simulink model "HighwayLaneChangeTestBench"  (R2022a)
settings: Solver=VariableStepAuto  StartTime=0.0  StopTime=inf  FixedStep=Ts  RelTol=1e-3
PostLoadFcn:
  | helperSLHighwayLaneChangeSetup;
undefined symbols (not defined in the file): actorProfiles, camera, DiscIntNeverNeededParam, driving, egoFrontExt, egoTTC, enableCCBehavior, enableLCBehavior, enableLCFBehavior, frontSafetyGap, latDevCost, mapInfo, matlabshared, maxAccel, maxCurvature, maxPlanningHorizon, maxYawRate, minVelocity, nextTTC, predictionHorizon, preferredLane, rearSafetyGap, replanRate, scenario, setSpeed, speedCost, targetFrontExt, timeCost, timeHorizon, timeResolution, Ts, u_max, u_min
libraries: drivingscenarioandsensors x8, rllib x1, sensorinslib x1, simulink x1
CloseFcn:
  | helperSLHighwayLaneChangeCleanUp;
settings Model: Creator=The MathWorks, Inc.  LastModifiedBy=leeju
settings SolverCC: ZeroCrossAlgorithm=Adaptive  AlgebraicLoopSolver=TrustRegion  MaxZcPerStep=1
settings DataIOCC: SaveOutput=off
settings DebuggingCC: MaskedZcDiagnostic=none  IgnoredZcDiagnostic=none  UnconnectedInputMsg=warning  UnconnectedOutputMsg=warning  UnconnectedLineMsg=warning  BusObjectLabelMismatch=none  SFMachineParentedDataDiag=warning
settings RTWCC: DLArmComputeVersion=19.05

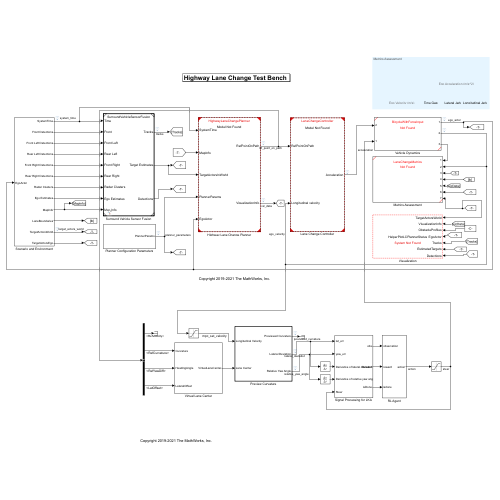
[thumbnail: Simulink's stored preview of the top-level diagram]
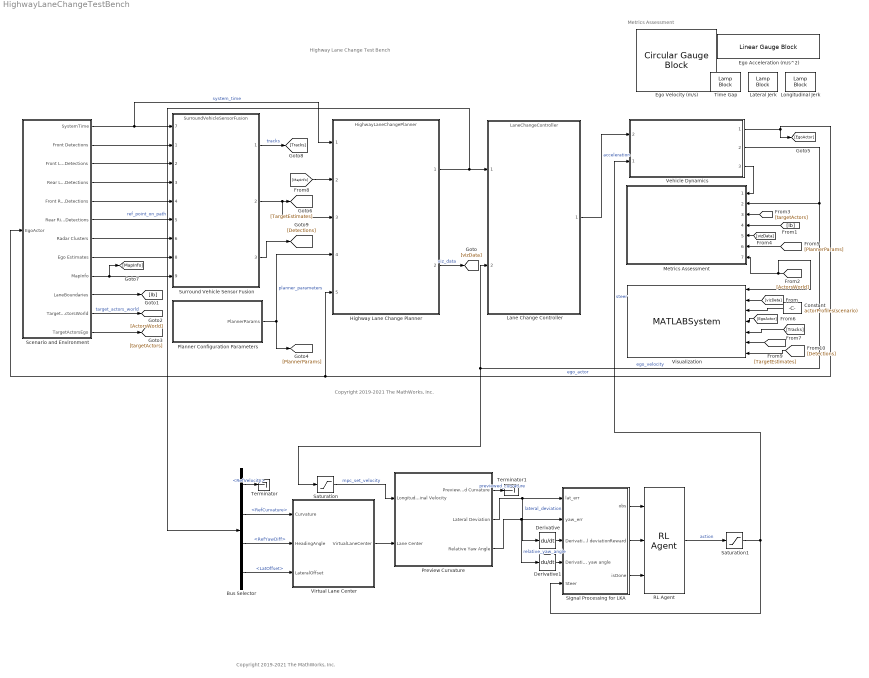
== system HighwayLaneChangeTestBench ==
  note: Copyright 2019-2021 The MathWorks, Inc.
  note: Metrics Assessment
  note: Highway Lane Change Test Bench
  note: Copyright 2019-2021 The MathWorks, Inc.
  Bus Selector : BusSelector  OutputSignals=RefVelocity,RefCurvature,RefYawDiff,LatOffset
  Constant : Constant  Value=actorProfiles(scenario)  OutDataTypeStr=Bus: BusActorProfiles
  Derivative : Derivative
  Derivative1 : Derivative
  Ego Acceleration (m/s^2) : LinearGaugeBlock  LabelPosition=Hide  ScaleMin=-5  ScaleMax=5
  Ego Velocity (m/s) : CircularGaugeBlock  LabelPosition=Hide  ScaleMax=50  TickInterval=5
  Highway Lane Change Planner : ModelReference  ModelNameDialog=HighwayLaneChangePlanner.slx  SimulationMode=Normal  ModelReferenceVersion=5.16
  Lane Change Controller : ModelReference  ModelNameDialog=LaneChangeController.slx  SimulationMode=Normal  ModelReferenceVersion=4.4
  Lateral Jerk : LampBlock  LabelPosition=Hide
  Longitudinal Jerk : LampBlock  LabelPosition=Hide
  Metrics Assessment : Subsystem  ReferencedSubsystem=LaneChangeMetrics
  Planner Configuration Parameters : Subsystem
  Preview Curvature : Subsystem  TreatAsAtomicUnit=on
  RL Agent : rllib/RL Agent  Agent=agent  ExternalActionAsInput=off  ProvideLastAction=off  ProvideCumRwd=off  TreatAsDirectFeedthrough=on  UseStrictObservationDataTypes=off
  Saturation : Saturate  UpperLimit=inf  LowerLimit=0.0001
  Saturation1 : Saturate  UpperLimit=u_max  LowerLimit=u_min
  Scenario and Environment : Subsystem
  "Signal Processing for LKA " : Subsystem
  Surround Vehicle Sensor Fusion : ModelReference  ModelNameDialog=SurroundVehicleSensorFusion.slx  SimulationMode=Normal  ModelReferenceVersion=5.215
      settings: PortSchema="{\"entries\":[{\"content\":{\"sides\":[{\"content\":{\"connectorIds\":[\"In7\",\"In1\",\"In2\",\"In3\",\"In4\",\"In5\",\"In6\",\"In8\",\"In9\"]},\"type\":\"ConnectorPlacement.EquallySpacedRectSide\",\"uuid\":\"babc32b8-473b-4a04-b824-251f7900e603\"},{\"content\":{\"connectorIds\":[\"Out1\",\"Out2\",\"Out3\"],\"side\":\"RIGHT\"},\"type\":\"ConnectorPlacement.EquallySpacedRectSide\",\"uuid\":\"6521796d-8396-47d7-a507-be3f8604ea95\"},{\"content\":{\"connectorIds\":[],\"side\":\"TOP\"},\"type\":\"ConnectorPlacement.EquallySpacedRectSide\",\"uuid\":\"3afcd3a1-01f6-437b-a186-b4f18cfd5e31\"}]},\"type\":\"ConnectorPlacement.EquallySpacedConnector\",\"uuid\":\"2716b65b-56e0-49c3-bc67-2edcf12b2a8e\"}],\"packageUris\":[\"http://schema.mathworks.com/mf0/Connector/R2020b\"],\"version\":\"1.0\"}"
  Terminator : Terminator
  Terminator1 : Terminator
  Time Gap : LampBlock  LabelPosition=Hide
  Vehicle Dynamics : Subsystem  ReferencedSubsystem=BicycleWithForceInput
      settings: PortSchema="{\"entries\":[{\"content\":{\"sides\":[{\"content\":{\"connectorIds\":[\"In2\",\"In1\"]},\"type\":\"ConnectorPlacement.EquallySpacedRectSide\",\"uuid\":\"f63f66bc-f59a-4e63-885b-0681004bade6\"},{\"content\":{\"connectorIds\":[\"Out1\",\"Out2\",\"Out3\"],\"side\":\"RIGHT\"},\"type\":\"ConnectorPlacement.EquallySpacedRectSide\",\"uuid\":\"8ac8ea57-0210-4a13-ad95-4f0a9335ab33\"},{\"content\":{\"connectorIds\":[],\"side\":\"TOP\"},\"type\":\"ConnectorPlacement.EquallySpacedRectSide\",\"uuid\":\"6d0b300d-41b2-47ad-8d2f-35db0d33cdc5\"}]},\"type\":\"ConnectorPlacement.EquallySpacedConnector\",\"uuid\":\"3215dd89-c688-4582-a904-15ea546ef61a\"}],\"packageUris\":[\"http://schema.mathworks.com/mf0/Connector/R2020b\"],\"version\":\"1.0\"}"
  Virtual Lane Center : Subsystem
  Visualization : MATLABSystem  System=HelperPlotLCPlannerStatus  ActorsInfo=Tracks  EnableTopView=on  EnableTrajTopView=on  EnableTracksTopView=on  EnableChaseView=on  EnableTrajChase=on  EnableCaplistChaseView=on  EnableTracksChaseView=on
      mask Type: HelperPlotLCPlannerStatus
      mask Display:
      | disp('HelperPlotLCPlannerStatus');
      | port_label('input',1,'TargetActorsWorld');
      | port_label('input',2,'VisualizationInfo');
      | port_label('input',3,'ObstacleProfiles');
      | port_label('input',4,'EgoActor');
      | port_label('input',5,'Tracks');
      | port_label('input',6,'EstimatedTargets');
      | port_label('input',7,'Detections');
  wires:
  Planner Configuration Parameters/1(PlannerParams) -> Highway Lane Change Planner/4, [PlannerParams]  "planner_parameters"
  Highway Lane Change Planner/2 -> [vizData]  "viz_data"
  Scenario and Environment/10(LaneBoundaries) -> [lb]
  [lb] -> Metrics Assessment/4
  Highway Lane Change Planner/1 -> Bus Selector/1, Lane Change Controller/1  "ref_point_on_path"
  [ActorsWorld] -> Metrics Assessment/7, Visualization/1
  Scenario and Environment/11(TargetActorsWorld) -> [ActorsWorld]  "target_actors_world"
  Scenario and Environment/12(TargetActorsEgo) -> [targetActors]
  [targetActors] -> Metrics Assessment/3
  Scenario and Environment/1(SystemTime) -> Highway Lane Change Planner/1, Surround Vehicle Sensor Fusion/7  "system_time"
  Vehicle Dynamics/1 -> Scenario and Environment/1(EgoActor), Highway Lane Change Planner/5, [EgoActor]  "ego_actor"
  Vehicle Dynamics/2 -> Saturation/1, Lane Change Controller/2, Metrics Assessment/2  "ego_velocity"
  Vehicle Dynamics/3 -> Metrics Assessment/1
  Lane Change Controller/1 -> Vehicle Dynamics/2  "acceleration"
  [vizData] -> Metrics Assessment/5
  [PlannerParams] -> Metrics Assessment/6
  Scenario and Environment/2(Front Detections) -> Surround Vehicle Sensor Fusion/1
  Scenario and Environment/3(Front Left Detections) -> Surround Vehicle Sensor Fusion/2
  Scenario and Environment/4(" Rear Left Detections") -> Surround Vehicle Sensor Fusion/3
  Scenario and Environment/5(Front Right Detections) -> Surround Vehicle Sensor Fusion/4
  Scenario and Environment/6(Rear Right Detections) -> Surround Vehicle Sensor Fusion/5
  Scenario and Environment/7(Radar Clusters) -> Surround Vehicle Sensor Fusion/6
  Scenario and Environment/8(Ego Estimates) -> Surround Vehicle Sensor Fusion/8
  [vizData] -> Visualization/2
  Constant/1 -> Visualization/3
  Scenario and Environment/9(MapInfo) -> Surround Vehicle Sensor Fusion/9, [MapInfo]
  [MapInfo] -> Highway Lane Change Planner/2
  Surround Vehicle Sensor Fusion/2 -> Highway Lane Change Planner/3, [TargetEstimates]
  Surround Vehicle Sensor Fusion/1 -> [Tracks]  "tracks"
  Surround Vehicle Sensor Fusion/3 -> [Detections]
  [Tracks] -> Visualization/5
  [Detections] -> Visualization/7
  [EgoActor] -> Visualization/4
  [TargetEstimates] -> Visualization/6
  Saturation1/1 -> "Signal Processing for LKA "/5(Steer), Vehicle Dynamics/1  "steer"
  Derivative1/1 -> "Signal Processing for LKA "/4(Derivative of relative yaw angle)
  "Signal Processing for LKA "/3(isDone) -> RL Agent/3
  "Signal Processing for LKA "/1(obs) -> RL Agent/1
  RL Agent/1 -> Saturation1/1  "action"
  "Signal Processing for LKA "/2(Reward) -> RL Agent/2
  Bus Selector/3 -> Virtual Lane Center/2(HeadingAngle)  "<RefYawDiff>"
  Saturation/1 -> Preview Curvature/1(Longitudinal Velocity)  "mpc_set_velocity"
  Virtual Lane Center/1(VirtualLaneCenter) -> Preview Curvature/2(Lane Center)
  Preview Curvature/3(Relative Yaw Angle) -> "Signal Processing for LKA "/2(yaw_err), Derivative1/1  "relative_yaw_angle"
  Bus Selector/2 -> Virtual Lane Center/1(Curvature)  "<RefCurvature>"
  Derivative/1 -> "Signal Processing for LKA "/3("Derivative of lateral deviation ")
  Bus Selector/4 -> Virtual Lane Center/3(LateralOffset)  "<LatOffset>"
  Preview Curvature/2(Lateral Deviation) -> "Signal Processing for LKA "/1(lat_err), Derivative/1  "lateral_deviation"
  Bus Selector/1 -> Terminator/1  "<RefVelocity>"
  Preview Curvature/1(Previewed Curvature) -> Terminator1/1  "previewed_curvature"

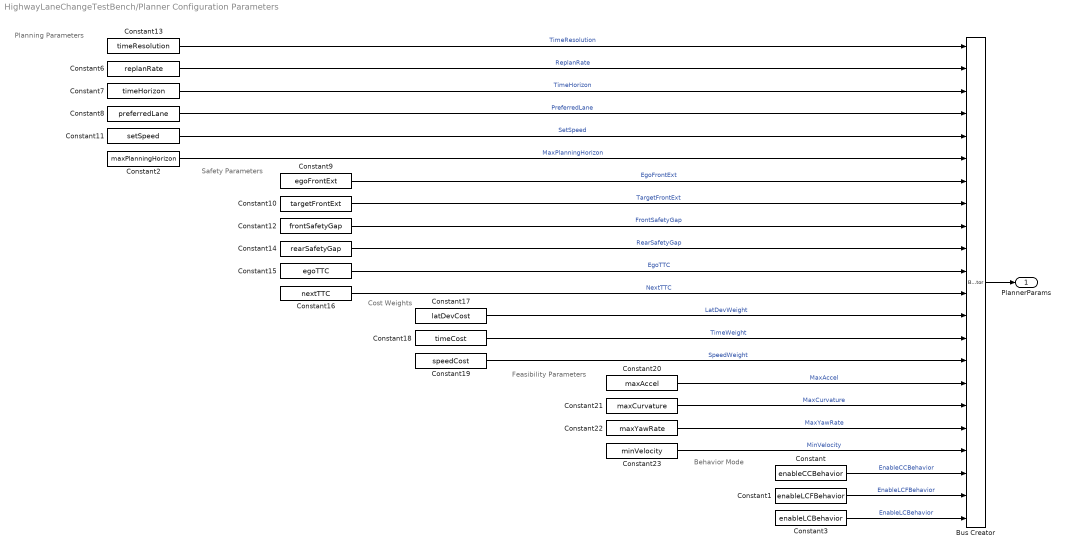
== system HighwayLaneChangeTestBench/Planner Configuration Parameters ==
  note: Planning Parameters
  note: Safety Parameters
  note: Cost Weights
  note: Feasibility Parameters
  note: Behavior Mode
  Bus Creator : BusCreator  Inputs=22  OutDataTypeStr=Bus: BusPlannerParams  NonVirtualBus=on
  Constant : Constant  Value=enableCCBehavior
  Constant1 : Constant  Value=enableLCFBehavior
  Constant10 : Constant  Value=targetFrontExt
  Constant11 : Constant  Value=setSpeed
  Constant12 : Constant  Value=frontSafetyGap
  Constant13 : Constant  Value=timeResolution
  Constant14 : Constant  Value=rearSafetyGap
  Constant15 : Constant  Value=egoTTC
  Constant16 : Constant  Value=nextTTC
  Constant17 : Constant  Value=latDevCost
  Constant18 : Constant  Value=timeCost
  Constant19 : Constant  Value=speedCost
  Constant2 : Constant  Value=maxPlanningHorizon
  Constant20 : Constant  Value=maxAccel
  Constant21 : Constant  Value=maxCurvature
  Constant22 : Constant  Value=maxYawRate
  Constant23 : Constant  Value=minVelocity
  Constant3 : Constant  Value=enableLCBehavior
  Constant6 : Constant  Value=replanRate
  Constant7 : Constant  Value=timeHorizon
  Constant8 : Constant  Value=preferredLane
  Constant9 : Constant  Value=egoFrontExt
  PlannerParams : Outport  OutDataTypeStr=Bus: BusPlannerParams
  wires:
  Constant19/1 -> Bus Creator/15  "SpeedWeight"
  Constant15/1 -> Bus Creator/11  "EgoTTC"
  Constant12/1 -> Bus Creator/9  "FrontSafetyGap"
  Constant6/1 -> Bus Creator/2  "ReplanRate"
  Constant14/1 -> Bus Creator/10  "RearSafetyGap"
  Constant20/1 -> Bus Creator/16  "MaxAccel"
  Constant18/1 -> Bus Creator/14  "TimeWeight"
  Constant11/1 -> Bus Creator/5  "SetSpeed"
  Constant13/1 -> Bus Creator/1  "TimeResolution"
  Constant23/1 -> Bus Creator/19  "MinVelocity"
  Constant9/1 -> Bus Creator/7  "EgoFrontExt"
  Constant16/1 -> Bus Creator/12  "NextTTC"
  Constant10/1 -> Bus Creator/8  "TargetFrontExt"
  Constant7/1 -> Bus Creator/3  "TimeHorizon"
  Constant21/1 -> Bus Creator/17  "MaxCurvature"
  Constant8/1 -> Bus Creator/4  "PreferredLane"
  Constant17/1 -> Bus Creator/13  "LatDevWeight"
  Bus Creator/1 -> PlannerParams/1
  Constant22/1 -> Bus Creator/18  "MaxYawRate"
  Constant/1 -> Bus Creator/20  "EnableCCBehavior"
  Constant1/1 -> Bus Creator/21  "EnableLCFBehavior"
  Constant3/1 -> Bus Creator/22  "EnableLCBehavior"
  Constant2/1 -> Bus Creator/6  "MaxPlanningHorizon"

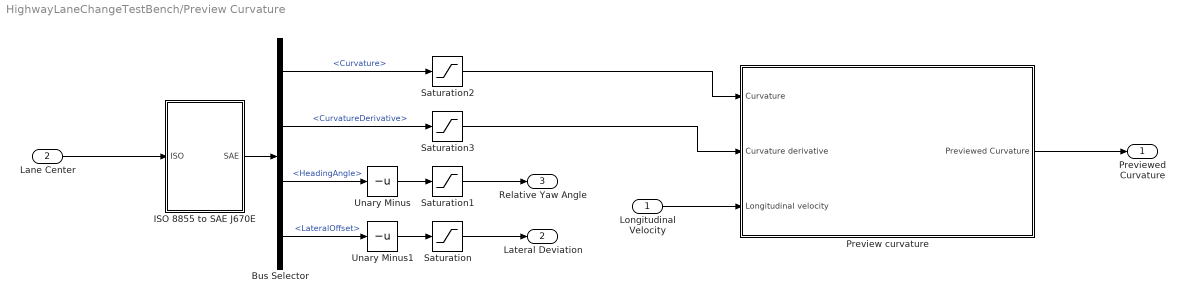
== system HighwayLaneChangeTestBench/Preview Curvature ==
  Longitudinal Velocity : Inport
  Lane Center : Inport  Port=2
  Bus Selector : BusSelector  OutputSignals=Curvature,CurvatureDerivative,HeadingAngle,LateralOffset
  ISO 8855 to SAE J670E : Subsystem
  Preview curvature : Subsystem
  Saturation : Saturate
  Saturation1 : Saturate  UpperLimit=0.8  LowerLimit=-0.8
  Saturation2 : Saturate  UpperLimit=0.15  LowerLimit=-0.15
  Saturation3 : Saturate  UpperLimit=0.06  LowerLimit=-0.06
  Unary Minus : UnaryMinus
  Unary Minus1 : UnaryMinus
  Previewed Curvature : Outport  VectorParamsAs1DForOutWhenUnconnected=off
  Lateral Deviation : Outport  Port=2  VectorParamsAs1DForOutWhenUnconnected=off
  Relative Yaw Angle : Outport  Port=3  VectorParamsAs1DForOutWhenUnconnected=off
  wires:
  Bus Selector/4 -> Unary Minus1/1  "<LateralOffset>"
  ISO 8855 to SAE J670E/1(SAE) -> Bus Selector/1
  Unary Minus1/1 -> Saturation/1
  Saturation3/1 -> Preview curvature/2(Curvature derivative)
  Bus Selector/1 -> Saturation2/1  "<Curvature>"
  Unary Minus/1 -> Saturation1/1
  Lane Center/1 -> ISO 8855 to SAE J670E/1(ISO)
  Saturation1/1 -> Relative Yaw Angle/1
  Longitudinal Velocity/1 -> Preview curvature/3(Longitudinal velocity)
  Saturation/1 -> Lateral Deviation/1
  Bus Selector/3 -> Unary Minus/1  "<HeadingAngle>"
  Saturation2/1 -> Preview curvature/1(Curvature)
  Bus Selector/2 -> Saturation3/1  "<CurvatureDerivative>"
  Preview curvature/1(Previewed Curvature) -> Previewed Curvature/1

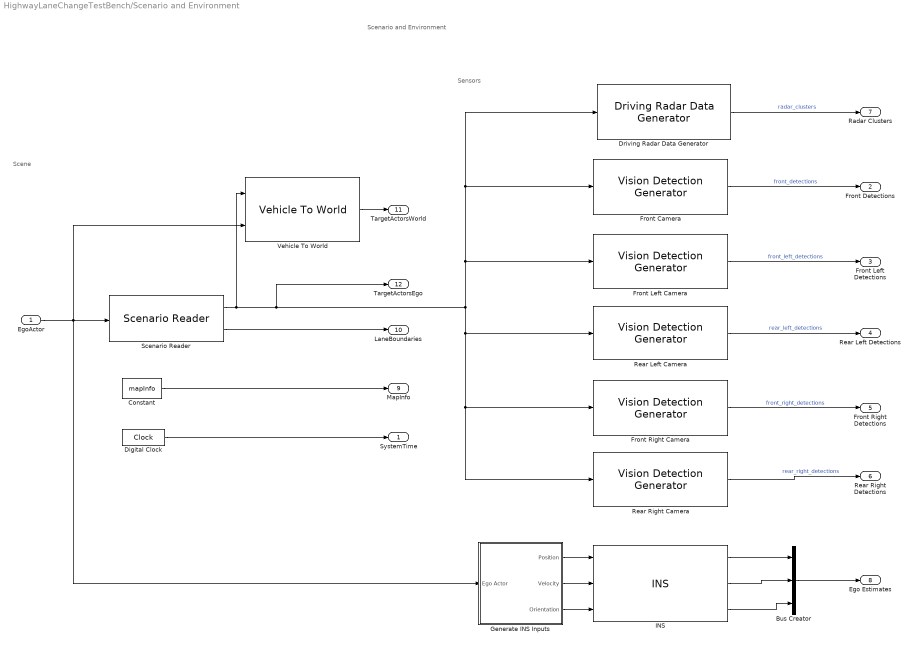
== system HighwayLaneChangeTestBench/Scenario and Environment ==
  note: Sensors
  note: Scene
  note: Scenario and Environment
  EgoActor : Inport
  Bus Creator : BusCreator  Inputs=3
  Constant : Constant  Value=mapInfo  OutDataTypeStr=Bus: BusMapInfo
  Digital Clock : DigitalClock  SampleTime=Ts
  Driving Radar Data Generator : drivingscenarioandsensors/Driving Radar Data Generator  SensorIndex=1  UpdateRate=10  MountingLocation=radar.Position  MountingAngles=radar.Rotation  HasElevation=off  HasRangeRate=on  HasNoise=on  HasFalseAlarms=off  HasOcclusion=off  MaxNumReportsSource=Property  MaxNumReports=50  TargetReportFormat=Clustered detections  DetectionCoordinates=Sensor spherical  TrackCoordinates=Body  BusNameSource=Property  BusName=BusDrivingRadarDataGenerator  AzimuthResolution=4  ElevationResolution=5  RangeResolution=2.5  RangeRateResolution=0.5  AzimuthBiasFraction=0.1  ElevationBiasFraction=0.1  RangeBiasFraction=0.05  RangeRateBiasFraction=0.05  FieldOfView=radar.FieldOfView  RangeLimits=radar.DetectionRanges  RangeRateLimits=[ -100, 100 ]  DetectionProbability=1  FalseAlarmRate=1e-06  ReferenceRange=100  ReferenceRCS=10  CenterFrequency=77e9  FilterInitializationFcn=initcvekf  ConfirmationThreshold=[2 3]  DeletionThreshold=[5 5]  InitialSeedSource=Repeatable  InitialSeed=0  UsedSeed=matlabshared.tracking.internal.SimulinkUtilities.seedManager(gcb)  ProfilesSource=From Scenario Reader block  ProfilesParameters=driving.internal.ActorProfilesRadarParameters  ProfilesExpression=struct('ClassID',0,'Length',4.7,'Width',1.8,'Height',1.4,'OriginOffset',[-1.35 0 0],'RCSPattern',[10 10;10 10],'RCSAzimuthAngles',[-180 180],'RCSElevationAngles',[-90 90])
      settings: SourceProductBaseCode=DR
  "Front Camera " : drivingscenarioandsensors/Vision Detection Generator  SensorIndex=2  DetectorOutput=Objects only  UpdateInterval=0.05  LaneUpdateInterval=0.1  SensorLocation=camera(1).Position(1:2)  Height=camera(1).Position(3)  Yaw=camera(1).Rotation(3)  Pitch=camera(1).Rotation(2)  Roll=camera(1).Rotation(1)  BusNameSource=Auto  BusName=BusObjectDetections  BusName2Source=Auto  BusName2=BusLaneDetections  MaxNumDetectionsSource=Property  MaxNumDetections=20  MaxNumLanesSource=Property  MaxNumLanes=30  DetectionCoordinates=Ego Cartesian  SimulateUsing=Interpreted execution  MaxRange=camera(1).DetectionRanges(2)  BoundingBoxAccuracy=1  ProcessNoiseIntensity=1  MaxSpeed=50  MaxAllowedOcclusion=0.99  MinObjectImageSize=[6 6]  DetectionProbability=0.95  FalsePositivesPerImage=0.02  MinLaneImageSize=[20 3]  LaneBoundaryAccuracy=3  HasNoise=off  InitialSeedSource=Specify seed  InitialSeed=0  UsedSeed=0  ActorProfilesSource=From Scenario Reader block  ActorProfilesParameters=driving.internal.ActorProfilesParameters  ActorProfilesExpression=[struct('ActorID',1,'ClassID',1,'Length',4.7,'Width',1.8,'Height',1.4,'OriginOffset',[-1.35 0 0],'MeshVertices',[3.7 -0.9 1.4;3.7 0.9 1.4;-1 0.9 1.4;-1 -0.9 1.4;3.7 -0.9 0;3.7 0.9 0;-1 0.9 0;-1 -0.9 0],'MeshFaces',[6 2 1;1 5 6;8 4 3;3 7 8;6 7 3;3 2 6;5 1 4;4 8 5;4 1 2;2 3 4;7 6 5;5 8 7],'RCSPattern',[10 10;10 10],'RCSAzimuthAngles',[-180 180],'RCSElevationAngles',[-90 90]); struct('ActorID',2,'ClassID',1,'Length',4.7,'Width',1.8,'Height',1.4,'OriginOffset',[-1.35 0 0],'MeshVertices',[3.7 -0.9 1.4;3.7 0.9 1.4;-1 0.9 1.4;-1 -0.9 1.4;3.7 -0.9 0;3.7 0.9 0;-1 0.9 0;-1 -0.9 0],'MeshFaces',[6 2 1;1 5 6;8 4 3;3 7 8;6 7 3;3 2 6;5 1 4;4 8 5;4 1 2;2 3 4;7 6 5;5 8 7],'RCSPattern',[10 10;10 10],'RCSAzimuthAngles',[-180 180],'RCSElevationAngles',[-90 90]); struct('ActorID',3,'ClassID',1,'Length',4.7,'Width',1.8,'Height',1.4,'OriginOffset',[-1.35 0 0],'MeshVertices',[3.7 -0.9 1.4;3.7 0.9 1.4;-1 0.9 1.4;-1 -0.9 1.4;3.7 -0.9 0;3.7 0.9 0;-1 0.9 0;-1 -0.9 0],'MeshFaces',[6 2 1;1 5 6;8 4 3;3 7 8;6 7 3;3 2 6;5 1 4;4 8 5;4 1 2;2 3 4;7 6 5;5 8 7],'RCSPattern',[10 10;10 10],'RCSAzimuthAngles',[-180 180],'RCSElevationAngles',[-90 90]); struct('ActorID',4,'ClassID',1,'Length',4.7,'Width',1.8,'Height',1.4,'OriginOffset',[-1.35 0 0],'MeshVertices',[3.7 -0.9 1.4;3.7 0.9 1.4;-1 0.9 1.4;-1 -0.9 1.4;3.7 -0.9 0;3.7 0.9 0;-1 0.9 0;-1 -0.9 0],'MeshFaces',[6 2 1;1 5 6;8 4 3;3 7 8;6 7 3;3 2 6;5 1 4;4 8 5;4 1 2;2 3 4;7 6 5;5 8 7],'RCSPattern',[10 10;10 10],'RCSAzimuthAngles',[-180 180],'RCSElevationAngles',[-90 90])]  Intrinsics=driving.internal.cameraIntrinsics('FocalLength',camera(1).FocalLength,'PrincipalPoint',camera(1).PrincipalPoint,'ImageSize',camera(1).ImageSize,'RadialDistortion',[0 0],'TangentialDistortion',[0 0],'Skew',0)
  Front Left Camera : drivingscenarioandsensors/Vision Detection Generator  SensorIndex=3  DetectorOutput=Objects only  UpdateInterval=0.05  LaneUpdateInterval=0.1  SensorLocation=camera(2).Position(1:2)  Height=camera(2).Position(3)  Yaw=camera(2).Rotation(3)  Pitch=camera(2).Rotation(2)  Roll=camera(2).Rotation(1)  BusNameSource=Auto  BusName=BusObjectDetections  BusName2Source=Auto  BusName2=BusLaneDetections  MaxNumDetectionsSource=Property  MaxNumDetections=20  MaxNumLanesSource=Property  MaxNumLanes=30  DetectionCoordinates=Ego Cartesian  SimulateUsing=Interpreted execution  MaxRange=camera(2).DetectionRanges(2)  BoundingBoxAccuracy=1  ProcessNoiseIntensity=1  MaxSpeed=50  MaxAllowedOcclusion=0.99  MinObjectImageSize=[6 6]  DetectionProbability=0.96  FalsePositivesPerImage=0.02  MinLaneImageSize=[20 3]  LaneBoundaryAccuracy=3  HasNoise=off  InitialSeedSource=Specify seed  InitialSeed=0.1  UsedSeed=0  ActorProfilesSource=From Scenario Reader block  ActorProfilesParameters=driving.internal.ActorProfilesParameters  ActorProfilesExpression=[struct('ActorID',1,'ClassID',1,'Length',4.7,'Width',1.8,'Height',1.4,'OriginOffset',[-1.35 0 0],'MeshVertices',[3.7 -0.9 1.4;3.7 0.9 1.4;-1 0.9 1.4;-1 -0.9 1.4;3.7 -0.9 0;3.7 0.9 0;-1 0.9 0;-1 -0.9 0],'MeshFaces',[6 2 1;1 5 6;8 4 3;3 7 8;6 7 3;3 2 6;5 1 4;4 8 5;4 1 2;2 3 4;7 6 5;5 8 7],'RCSPattern',[10 10;10 10],'RCSAzimuthAngles',[-180 180],'RCSElevationAngles',[-90 90]); struct('ActorID',2,'ClassID',1,'Length',4.7,'Width',1.8,'Height',1.4,'OriginOffset',[-1.35 0 0],'MeshVertices',[3.7 -0.9 1.4;3.7 0.9 1.4;-1 0.9 1.4;-1 -0.9 1.4;3.7 -0.9 0;3.7 0.9 0;-1 0.9 0;-1 -0.9 0],'MeshFaces',[6 2 1;1 5 6;8 4 3;3 7 8;6 7 3;3 2 6;5 1 4;4 8 5;4 1 2;2 3 4;7 6 5;5 8 7],'RCSPattern',[10 10;10 10],'RCSAzimuthAngles',[-180 180],'RCSElevationAngles',[-90 90]); struct('ActorID',3,'ClassID',1,'Length',4.7,'Width',1.8,'Height',1.4,'OriginOffset',[-1.35 0 0],'MeshVertices',[3.7 -0.9 1.4;3.7 0.9 1.4;-1 0.9 1.4;-1 -0.9 1.4;3.7 -0.9 0;3.7 0.9 0;-1 0.9 0;-1 -0.9 0],'MeshFaces',[6 2 1;1 5 6;8 4 3;3 7 8;6 7 3;3 2 6;5 1 4;4 8 5;4 1 2;2 3 4;7 6 5;5 8 7],'RCSPattern',[10 10;10 10],'RCSAzimuthAngles',[-180 180],'RCSElevationAngles',[-90 90]); struct('ActorID',4,'ClassID',1,'Length',4.7,'Width',1.8,'Height',1.4,'OriginOffset',[-1.35 0 0],'MeshVertices',[3.7 -0.9 1.4;3.7 0.9 1.4;-1 0.9 1.4;-1 -0.9 1.4;3.7 -0.9 0;3.7 0.9 0;-1 0.9 0;-1 -0.9 0],'MeshFaces',[6 2 1;1 5 6;8 4 3;3 7 8;6 7 3;3 2 6;5 1 4;4 8 5;4 1 2;2 3 4;7 6 5;5 8 7],'RCSPattern',[10 10;10 10],'RCSAzimuthAngles',[-180 180],'RCSElevationAngles',[-90 90])]  Intrinsics=driving.internal.cameraIntrinsics('FocalLength',camera(2).FocalLength,'PrincipalPoint',camera(2).PrincipalPoint,'ImageSize',camera(2).ImageSize,'RadialDistortion',[0 0],'TangentialDistortion',[0 0],'Skew',0)
  Front Right Camera : drivingscenarioandsensors/Vision Detection Generator  SensorIndex=5  DetectorOutput=Objects only  UpdateInterval=0.05  LaneUpdateInterval=0.1  SensorLocation=camera(4).Position(1:2)  Height=camera(4).Position(3)  Yaw=camera(4).Rotation(3)  Pitch=camera(4).Rotation(2)  Roll=camera(4).Rotation(1)  BusNameSource=Auto  BusName=BusObjectDetections  BusName2Source=Auto  BusName2=BusLaneDetections  MaxNumDetectionsSource=Property  MaxNumDetections=20  MaxNumLanesSource=Property  MaxNumLanes=30  DetectionCoordinates=Ego Cartesian  SimulateUsing=Interpreted execution  MaxRange=camera(4).DetectionRanges(2)  BoundingBoxAccuracy=1  ProcessNoiseIntensity=1  MaxSpeed=50  MaxAllowedOcclusion=0.99  MinObjectImageSize=[6 6]  DetectionProbability=0.96  FalsePositivesPerImage=0.02  MinLaneImageSize=[20 3]  LaneBoundaryAccuracy=3  HasNoise=off  InitialSeedSource=Specify seed  InitialSeed=0.3  UsedSeed=0  ActorProfilesSource=From Scenario Reader block  ActorProfilesParameters=driving.internal.ActorProfilesParameters  ActorProfilesExpression=[struct('ActorID',1,'ClassID',1,'Length',4.7,'Width',1.8,'Height',1.4,'OriginOffset',[-1.35 0 0],'MeshVertices',[3.7 -0.9 1.4;3.7 0.9 1.4;-1 0.9 1.4;-1 -0.9 1.4;3.7 -0.9 0;3.7 0.9 0;-1 0.9 0;-1 -0.9 0],'MeshFaces',[6 2 1;1 5 6;8 4 3;3 7 8;6 7 3;3 2 6;5 1 4;4 8 5;4 1 2;2 3 4;7 6 5;5 8 7],'RCSPattern',[10 10;10 10],'RCSAzimuthAngles',[-180 180],'RCSElevationAngles',[-90 90]); struct('ActorID',2,'ClassID',1,'Length',4.7,'Width',1.8,'Height',1.4,'OriginOffset',[-1.35 0 0],'MeshVertices',[3.7 -0.9 1.4;3.7 0.9 1.4;-1 0.9 1.4;-1 -0.9 1.4;3.7 -0.9 0;3.7 0.9 0;-1 0.9 0;-1 -0.9 0],'MeshFaces',[6 2 1;1 5 6;8 4 3;3 7 8;6 7 3;3 2 6;5 1 4;4 8 5;4 1 2;2 3 4;7 6 5;5 8 7],'RCSPattern',[10 10;10 10],'RCSAzimuthAngles',[-180 180],'RCSElevationAngles',[-90 90]); struct('ActorID',3,'ClassID',1,'Length',4.7,'Width',1.8,'Height',1.4,'OriginOffset',[-1.35 0 0],'MeshVertices',[3.7 -0.9 1.4;3.7 0.9 1.4;-1 0.9 1.4;-1 -0.9 1.4;3.7 -0.9 0;3.7 0.9 0;-1 0.9 0;-1 -0.9 0],'MeshFaces',[6 2 1;1 5 6;8 4 3;3 7 8;6 7 3;3 2 6;5 1 4;4 8 5;4 1 2;2 3 4;7 6 5;5 8 7],'RCSPattern',[10 10;10 10],'RCSAzimuthAngles',[-180 180],'RCSElevationAngles',[-90 90]); struct('ActorID',4,'ClassID',1,'Length',4.7,'Width',1.8,'Height',1.4,'OriginOffset',[-1.35 0 0],'MeshVertices',[3.7 -0.9 1.4;3.7 0.9 1.4;-1 0.9 1.4;-1 -0.9 1.4;3.7 -0.9 0;3.7 0.9 0;-1 0.9 0;-1 -0.9 0],'MeshFaces',[6 2 1;1 5 6;8 4 3;3 7 8;6 7 3;3 2 6;5 1 4;4 8 5;4 1 2;2 3 4;7 6 5;5 8 7],'RCSPattern',[10 10;10 10],'RCSAzimuthAngles',[-180 180],'RCSElevationAngles',[-90 90])]  Intrinsics=driving.internal.cameraIntrinsics('FocalLength',camera(4).FocalLength,'PrincipalPoint',camera(4).PrincipalPoint,'ImageSize',camera(4).ImageSize,'RadialDistortion',[0 0],'TangentialDistortion',[0 0],'Skew',0)
  Generate INS Inputs : Subsystem  TreatAsAtomicUnit=on
  INS : sensorinslib/INS  MountingLocation=[0 0 0]  RollAccuracy=0.1  PitchAccuracy=0.1  YawAccuracy=0.1  PositionAccuracy=0.1  VelocityAccuracy=0.1  UseAccelAndAngVel=off  AccelerationAccuracy=0  AngularVelocityAccuracy=0  TimeInput=off  PositionErrorFactor=[0 0 0]  SeedDouble=67  SimulateUsing=Interpreted execution
      settings: SourceProductBaseCode=TF,DR,NV,UV
  Rear Left Camera : drivingscenarioandsensors/Vision Detection Generator  SensorIndex=4  DetectorOutput=Objects only  UpdateInterval=0.05  LaneUpdateInterval=0.1  SensorLocation=camera(3).Position(1:2)  Height=camera(3).Position(3)  Yaw=camera(3).Rotation(3)  Pitch=camera(3).Rotation(2)  Roll=camera(3).Rotation(1)  BusNameSource=Auto  BusName=BusObjectDetections  BusName2Source=Auto  BusName2=BusLaneDetections  MaxNumDetectionsSource=Property  MaxNumDetections=20  MaxNumLanesSource=Property  MaxNumLanes=30  DetectionCoordinates=Ego Cartesian  SimulateUsing=Interpreted execution  MaxRange=camera(3).DetectionRanges(2)  BoundingBoxAccuracy=1  ProcessNoiseIntensity=1  MaxSpeed=50  MaxAllowedOcclusion=0.99  MinObjectImageSize=[6 6]  DetectionProbability=0.95  FalsePositivesPerImage=0.02  MinLaneImageSize=[20 3]  LaneBoundaryAccuracy=3  HasNoise=off  InitialSeedSource=Specify seed  InitialSeed=0.2  UsedSeed=0  ActorProfilesSource=From Scenario Reader block  ActorProfilesParameters=driving.internal.ActorProfilesParameters  ActorProfilesExpression=[struct('ActorID',1,'ClassID',1,'Length',4.7,'Width',1.8,'Height',1.4,'OriginOffset',[-1.35 0 0],'MeshVertices',[3.7 -0.9 1.4;3.7 0.9 1.4;-1 0.9 1.4;-1 -0.9 1.4;3.7 -0.9 0;3.7 0.9 0;-1 0.9 0;-1 -0.9 0],'MeshFaces',[6 2 1;1 5 6;8 4 3;3 7 8;6 7 3;3 2 6;5 1 4;4 8 5;4 1 2;2 3 4;7 6 5;5 8 7],'RCSPattern',[10 10;10 10],'RCSAzimuthAngles',[-180 180],'RCSElevationAngles',[-90 90]); struct('ActorID',2,'ClassID',1,'Length',4.7,'Width',1.8,'Height',1.4,'OriginOffset',[-1.35 0 0],'MeshVertices',[3.7 -0.9 1.4;3.7 0.9 1.4;-1 0.9 1.4;-1 -0.9 1.4;3.7 -0.9 0;3.7 0.9 0;-1 0.9 0;-1 -0.9 0],'MeshFaces',[6 2 1;1 5 6;8 4 3;3 7 8;6 7 3;3 2 6;5 1 4;4 8 5;4 1 2;2 3 4;7 6 5;5 8 7],'RCSPattern',[10 10;10 10],'RCSAzimuthAngles',[-180 180],'RCSElevationAngles',[-90 90]); struct('ActorID',3,'ClassID',1,'Length',4.7,'Width',1.8,'Height',1.4,'OriginOffset',[-1.35 0 0],'MeshVertices',[3.7 -0.9 1.4;3.7 0.9 1.4;-1 0.9 1.4;-1 -0.9 1.4;3.7 -0.9 0;3.7 0.9 0;-1 0.9 0;-1 -0.9 0],'MeshFaces',[6 2 1;1 5 6;8 4 3;3 7 8;6 7 3;3 2 6;5 1 4;4 8 5;4 1 2;2 3 4;7 6 5;5 8 7],'RCSPattern',[10 10;10 10],'RCSAzimuthAngles',[-180 180],'RCSElevationAngles',[-90 90]); struct('ActorID',4,'ClassID',1,'Length',4.7,'Width',1.8,'Height',1.4,'OriginOffset',[-1.35 0 0],'MeshVertices',[3.7 -0.9 1.4;3.7 0.9 1.4;-1 0.9 1.4;-1 -0.9 1.4;3.7 -0.9 0;3.7 0.9 0;-1 0.9 0;-1 -0.9 0],'MeshFaces',[6 2 1;1 5 6;8 4 3;3 7 8;6 7 3;3 2 6;5 1 4;4 8 5;4 1 2;2 3 4;7 6 5;5 8 7],'RCSPattern',[10 10;10 10],'RCSAzimuthAngles',[-180 180],'RCSElevationAngles',[-90 90])]  Intrinsics=driving.internal.cameraIntrinsics('FocalLength',camera(3).FocalLength,'PrincipalPoint',camera(3).PrincipalPoint,'ImageSize',camera(3).ImageSize,'RadialDistortion',[0 0],'TangentialDistortion',[0 0],'Skew',0)
  Rear Right Camera : drivingscenarioandsensors/Vision Detection Generator  SensorIndex=6  DetectorOutput=Objects only  UpdateInterval=0.05  LaneUpdateInterval=0.1  SensorLocation=camera(5).Position(1:2)  Height=camera(5).Position(3)  Yaw=camera(5).Rotation(3)  Pitch=camera(5).Rotation(2)  Roll=camera(5).Rotation(1)  BusNameSource=Auto  BusName=BusObjectDetections  BusName2Source=Auto  BusName2=BusLaneDetections  MaxNumDetectionsSource=Property  MaxNumDetections=20  MaxNumLanesSource=Property  MaxNumLanes=30  DetectionCoordinates=Ego Cartesian  SimulateUsing=Interpreted execution  MaxRange=camera(5).DetectionRanges(2)  BoundingBoxAccuracy=1  ProcessNoiseIntensity=1  MaxSpeed=50  MaxAllowedOcclusion=0.99  MinObjectImageSize=[6 6]  DetectionProbability=0.95  FalsePositivesPerImage=0.02  MinLaneImageSize=[20 3]  LaneBoundaryAccuracy=3  HasNoise=off  InitialSeedSource=Specify seed  InitialSeed=0.4  UsedSeed=0  ActorProfilesSource=From Scenario Reader block  ActorProfilesParameters=driving.internal.ActorProfilesParameters  ActorProfilesExpression=[struct('ActorID',1,'ClassID',1,'Length',4.7,'Width',1.8,'Height',1.4,'OriginOffset',[-1.35 0 0],'MeshVertices',[3.7 -0.9 1.4;3.7 0.9 1.4;-1 0.9 1.4;-1 -0.9 1.4;3.7 -0.9 0;3.7 0.9 0;-1 0.9 0;-1 -0.9 0],'MeshFaces',[6 2 1;1 5 6;8 4 3;3 7 8;6 7 3;3 2 6;5 1 4;4 8 5;4 1 2;2 3 4;7 6 5;5 8 7],'RCSPattern',[10 10;10 10],'RCSAzimuthAngles',[-180 180],'RCSElevationAngles',[-90 90]); struct('ActorID',2,'ClassID',1,'Length',4.7,'Width',1.8,'Height',1.4,'OriginOffset',[-1.35 0 0],'MeshVertices',[3.7 -0.9 1.4;3.7 0.9 1.4;-1 0.9 1.4;-1 -0.9 1.4;3.7 -0.9 0;3.7 0.9 0;-1 0.9 0;-1 -0.9 0],'MeshFaces',[6 2 1;1 5 6;8 4 3;3 7 8;6 7 3;3 2 6;5 1 4;4 8 5;4 1 2;2 3 4;7 6 5;5 8 7],'RCSPattern',[10 10;10 10],'RCSAzimuthAngles',[-180 180],'RCSElevationAngles',[-90 90]); struct('ActorID',3,'ClassID',1,'Length',4.7,'Width',1.8,'Height',1.4,'OriginOffset',[-1.35 0 0],'MeshVertices',[3.7 -0.9 1.4;3.7 0.9 1.4;-1 0.9 1.4;-1 -0.9 1.4;3.7 -0.9 0;3.7 0.9 0;-1 0.9 0;-1 -0.9 0],'MeshFaces',[6 2 1;1 5 6;8 4 3;3 7 8;6 7 3;3 2 6;5 1 4;4 8 5;4 1 2;2 3 4;7 6 5;5 8 7],'RCSPattern',[10 10;10 10],'RCSAzimuthAngles',[-180 180],'RCSElevationAngles',[-90 90]); struct('ActorID',4,'ClassID',1,'Length',4.7,'Width',1.8,'Height',1.4,'OriginOffset',[-1.35 0 0],'MeshVertices',[3.7 -0.9 1.4;3.7 0.9 1.4;-1 0.9 1.4;-1 -0.9 1.4;3.7 -0.9 0;3.7 0.9 0;-1 0.9 0;-1 -0.9 0],'MeshFaces',[6 2 1;1 5 6;8 4 3;3 7 8;6 7 3;3 2 6;5 1 4;4 8 5;4 1 2;2 3 4;7 6 5;5 8 7],'RCSPattern',[10 10;10 10],'RCSAzimuthAngles',[-180 180],'RCSElevationAngles',[-90 90])]  Intrinsics=driving.internal.cameraIntrinsics('FocalLength',camera(5).FocalLength,'PrincipalPoint',camera(5).PrincipalPoint,'ImageSize',camera(5).ImageSize,'RadialDistortion',[0 0],'TangentialDistortion',[0 0],'Skew',0)
  Scenario Reader : drivingscenarioandsensors/Scenario Reader  ScenarioSource=From workspace  ScenarioFileName=CurevedRoadNetwork.mat  ScenarioVariableName=scenario  OutputCoordinateSystem=Vehicle coordinates  EgoVehicleSource=Input port  EgoVehicleActorID=egoInitialPose.ActorID  OrientVehiclesOnRoad=off  OutputEgoVehiclePose=off  OutputEgoVehicleState=off  SampleTime=0.1  LaneBoundaryOutput=Ego vehicle lane boundaries  LaneBoundaryDistance=0:0.5:60  LaneBoundaryLocation=Center of lane markings  BusNameSource=Property  BusName=BusActorsTruth  BusNumActorsSource=Scenario  BusNumActors=100  BusName2Source=Auto  BusName2=BusLaneBoundaries  BusNumLaneBoundariesSource=Scenario  BusNumLaneBoundaries=10  BusName3Source=Auto  BusName3=BusEgoActor  BusName4Source=Auto  BusName4=BusEgoState  ShowCoordinateLabels=on  SimulateUsing=Interpreted execution
  Vehicle To World : drivingscenarioandsensors/Vehicle To World  BusNameSource=Auto  BusName=BusVehicleToWorldActors  SimulateUsing=Interpreted execution
      settings: SourceProductBaseCode=DR
  SystemTime : Outport
  Front Detections : Outport  Port=2
  Front Left Detections : Outport  Port=3
  " Rear Left Detections" : Outport  Port=4
  Front Right Detections : Outport  Port=5
  Rear Right Detections : Outport  Port=6
  Radar Clusters : Outport  Port=7  OutDataTypeStr=Bus: BusDrivingRadarDataGenerator
  Ego Estimates : Outport  Port=8  OutDataTypeStr=Bus: BusEgoPose
  MapInfo : Outport  Port=9  OutDataTypeStr=Bus: BusMapInfo
  LaneBoundaries : Outport  Port=10
  TargetActorsWorld : Outport  Port=11  OutDataTypeStr=Bus: BusActorsTruth
  TargetActorsEgo : Outport  Port=12  OutDataTypeStr=Bus: BusActorsTruth
  wires:
  Scenario Reader/1 -> Driving Radar Data Generator/1, "Front Camera "/1, Front Left Camera/1, Rear Right Camera/1, Front Right Camera/1, Rear Left Camera/1, TargetActorsEgo/1, Vehicle To World/1
  Constant/1 -> MapInfo/1
  Digital Clock/1 -> SystemTime/1
  Rear Right Camera/1 -> Rear Right Detections/1  "rear_right_detections"
  Front Left Camera/1 -> Front Left Detections/1  "front_left_detections"
  Driving Radar Data Generator/1 -> Radar Clusters/1  "radar_clusters"
  Front Right Camera/1 -> Front Right Detections/1  "front_right_detections"
  Rear Left Camera/1 -> " Rear Left Detections"/1  "rear_left_detections"
  "Front Camera "/1 -> Front Detections/1  "front_detections"
  Scenario Reader/2 -> LaneBoundaries/1
  Vehicle To World/1 -> TargetActorsWorld/1
  INS/1 -> Bus Creator/1
  INS/3 -> Bus Creator/3
  EgoActor/1 -> Generate INS Inputs/1(Ego Actor), Vehicle To World/2, Scenario Reader/1
  Bus Creator/1 -> Ego Estimates/1
  INS/2 -> Bus Creator/2
  Generate INS Inputs/3(Orientation) -> INS/3
  Generate INS Inputs/2(Velocity) -> INS/2
  Generate INS Inputs/1(Position) -> INS/1

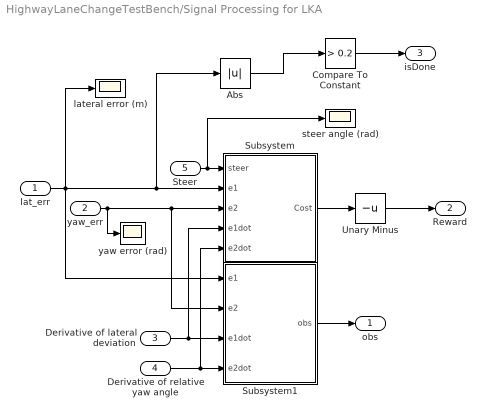
== system HighwayLaneChangeTestBench/Signal Processing for LKA  ==
  lat_err : Inport
  yaw_err : Inport  Port=2
  "Derivative of lateral deviation " : Inport  Port=3
  Derivative of relative yaw angle : Inport  Port=4
  Steer : Inport  Port=5
  Abs : Abs  SaturateOnIntegerOverflow=off
  Compare To Constant : simulink/Logic and Bit Operations/Compare To Constant  relop=>  const=0.2  OutDataTypeStr=boolean
  Subsystem : Subsystem
  Subsystem1 : Subsystem
  Unary Minus : UnaryMinus
  lateral error (m) : Scope
  "steer angle (rad) " : Scope
  yaw error (rad) : Scope
  obs : Outport  VectorParamsAs1DForOutWhenUnconnected=off
  Reward : Outport  Port=2  VectorParamsAs1DForOutWhenUnconnected=off
  isDone : Outport  Port=3  VectorParamsAs1DForOutWhenUnconnected=off
  wires:
  Subsystem/1(Cost) -> Unary Minus/1
  Unary Minus/1 -> Reward/1
  lat_err/1 -> Subsystem1/1(e1), Subsystem/2(e1), Abs/1, lateral error (m)/1
  yaw_err/1 -> yaw error (rad)/1, Subsystem1/2(e2), Subsystem/3(e2)
  Abs/1 -> Compare To Constant/1
  Compare To Constant/1 -> isDone/1
  Subsystem1/1(obs) -> obs/1
  "Derivative of lateral deviation "/1 -> Subsystem/4(e1dot), Subsystem1/3(e1dot)
  Derivative of relative yaw angle/1 -> Subsystem/5(e2dot), Subsystem1/4(e2dot)
  Steer/1 -> Subsystem/1(steer), "steer angle (rad) "/1

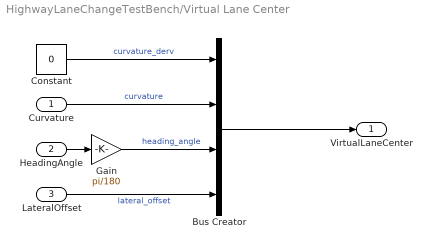
== system HighwayLaneChangeTestBench/Virtual Lane Center ==
  Curvature : Inport
  HeadingAngle : Inport  Port=2
  LateralOffset : Inport  Port=3
  Bus Creator : BusCreator  Inputs=4
  Constant : Constant  Value=0
  Gain : Gain  Gain=pi/180
  VirtualLaneCenter : Outport  VectorParamsAs1DForOutWhenUnconnected=off
  wires:
  Bus Creator/1 -> VirtualLaneCenter/1
  Gain/1 -> Bus Creator/3  "heading_angle"
  LateralOffset/1 -> Bus Creator/4  "lateral_offset"
  HeadingAngle/1 -> Gain/1
  Curvature/1 -> Bus Creator/2  "curvature"
  Constant/1 -> Bus Creator/1  "curvature_derv"

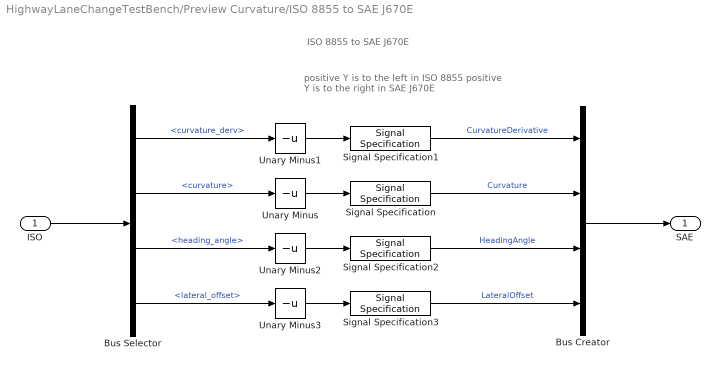
== system HighwayLaneChangeTestBench/Preview Curvature/ISO 8855 to SAE J670E ==
  note: positive Y is to the left in ISO 8855
      | positive Y is to the right in SAE J670E
  note: ISO 8855 to SAE J670E
  ISO : Inport
  Bus Creator : BusCreator  Inputs=4
  Bus Selector : BusSelector  OutputSignals=curvature_derv,curvature,heading_angle,lateral_offset
  Signal Specification : SignalSpecification  Unit=1/m
  Signal Specification1 : SignalSpecification  Unit=1/m^2
  Signal Specification2 : SignalSpecification  Unit=rad
  Signal Specification3 : SignalSpecification  Unit=m
  Unary Minus{,1..3} (4 alike) : UnaryMinus
  SAE : Outport  VectorParamsAs1DForOutWhenUnconnected=off
  wires:
  ISO/1 -> Bus Selector/1
  Bus Selector/2 -> Unary Minus/1  "<curvature>"
  Bus Selector/1 -> Unary Minus1/1  "<curvature_derv>"
  Bus Selector/3 -> Unary Minus2/1  "<heading_angle>"
  Bus Selector/4 -> Unary Minus3/1  "<lateral_offset>"
  Bus Creator/1 -> SAE/1
  Signal Specification/1 -> Bus Creator/2  "Curvature"
  Unary Minus1/1 -> Signal Specification1/1
  Unary Minus2/1 -> Signal Specification2/1
  Unary Minus3/1 -> Signal Specification3/1
  Unary Minus/1 -> Signal Specification/1
  Signal Specification1/1 -> Bus Creator/1  "CurvatureDerivative"
  Signal Specification2/1 -> Bus Creator/3  "HeadingAngle"
  Signal Specification3/1 -> Bus Creator/4  "LateralOffset"

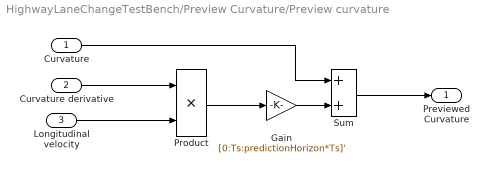
== system HighwayLaneChangeTestBench/Preview Curvature/Preview curvature ==
  Curvature : Inport
  Curvature derivative : Inport  Port=2
  Longitudinal velocity : Inport  Port=3
  Gain : Gain  Gain=[0:Ts:predictionHorizon*Ts]'
  Product : Product
  Sum : Sum
  Previewed Curvature : Outport  VectorParamsAs1DForOutWhenUnconnected=off
  wires:
  Sum/1 -> Previewed Curvature/1
  Curvature/1 -> Sum/1
  Gain/1 -> Sum/2
  Product/1 -> Gain/1
  Longitudinal velocity/1 -> Product/2
  Curvature derivative/1 -> Product/1

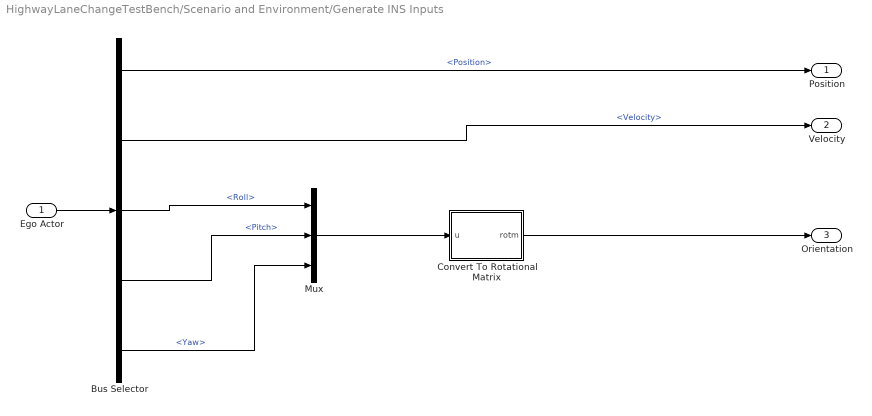
== system HighwayLaneChangeTestBench/Scenario and Environment/Generate INS Inputs ==
  Ego Actor : Inport
  Bus Selector : BusSelector  OutputSignals=Position,Velocity,Roll,Pitch,Yaw
  Convert To Rotational Matrix : MATLAB Function  TreatAsAtomicUnit=on
  Mux : Mux  Inputs=3
  Position : Outport
  Velocity : Outport  Port=2
  Orientation : Outport  Port=3
  wires:
  Bus Selector/2 -> Velocity/1  "<Velocity>"
  Bus Selector/1 -> Position/1  "<Position>"
  Bus Selector/5 -> Mux/3  "<Yaw>"
  Bus Selector/4 -> Mux/2  "<Pitch>"
  Bus Selector/3 -> Mux/1  "<Roll>"
  Ego Actor/1 -> Bus Selector/1
  Mux/1 -> Convert To Rotational Matrix/1(u)
  Convert To Rotational Matrix/1(rotm) -> Orientation/1

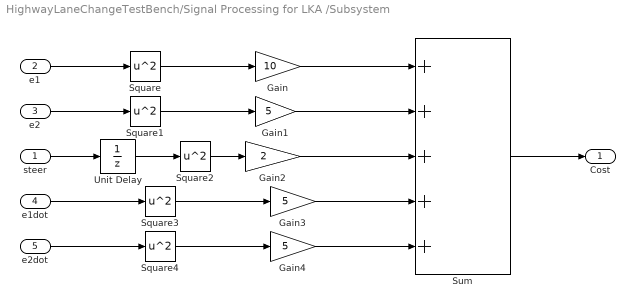
== system HighwayLaneChangeTestBench/Signal Processing for LKA /Subsystem ==
  steer : Inport
  e1 : Inport  Port=2
  e2 : Inport  Port=3
  e1dot : Inport  Port=4
  e2dot : Inport  Port=5
  Gain : Gain  Gain=10
  Gain1 : Gain  Gain=5
  Gain2 : Gain  Gain=2
  Gain3 : Gain  Gain=5
  Gain4 : Gain  Gain=5
  Square{,1..4} (5 alike) : Math  Operator=square  SignedPower=on
  Sum : Sum  Inputs=+++++
  Unit Delay : UnitDelay  SampleTime=-1  HasFrameUpgradeWarning=on
  Cost : Outport  VectorParamsAs1DForOutWhenUnconnected=off
  wires:
  Gain1/1 -> Sum/2
  e1/1 -> Square/1
  e2/1 -> Square1/1
  Sum/1 -> Cost/1
  Gain/1 -> Sum/1
  Square/1 -> Gain/1
  Square1/1 -> Gain1/1
  steer/1 -> Unit Delay/1
  Square2/1 -> Gain2/1
  Gain2/1 -> Sum/3
  Unit Delay/1 -> Square2/1
  Square3/1 -> Gain3/1
  Gain3/1 -> Sum/4
  e1dot/1 -> Square3/1
  e2dot/1 -> Square4/1
  Square4/1 -> Gain4/1
  Gain4/1 -> Sum/5

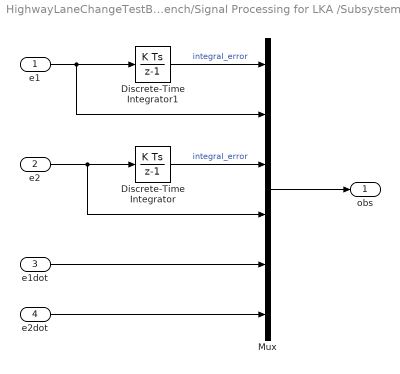
== system HighwayLaneChangeTestBench/Signal Processing for LKA /Subsystem1 ==
  e1 : Inport
  e2 : Inport  Port=2
  e1dot : Inport  Port=3
  e2dot : Inport  Port=4
  Discrete-Time Integrator : DiscreteIntegrator  SampleTime=-1  ICPrevOutput=DiscIntNeverNeededParam  ICPrevScaledInput=DiscIntNeverNeededParam
  Discrete-Time Integrator1 : DiscreteIntegrator  SampleTime=-1  ICPrevOutput=DiscIntNeverNeededParam  ICPrevScaledInput=DiscIntNeverNeededParam
  Mux : Mux  Inputs=6
  obs : Outport  VectorParamsAs1DForOutWhenUnconnected=off
  wires:
  e1/1 -> Mux/2, Discrete-Time Integrator1/1
  Mux/1 -> obs/1
  Discrete-Time Integrator1/1 -> Mux/1  "integral_error"
  e2/1 -> Mux/4, Discrete-Time Integrator/1
  Discrete-Time Integrator/1 -> Mux/3  "integral_error"
  e1dot/1 -> Mux/5
  e2dot/1 -> Mux/6

== matlab function HighwayLaneChangeTestBench/Scenario and Environment/Generate INS Inputs/Convert To Rotational Matrix ==
  data: u input; rotm output size=[3 3]
function rotm = eul2rotMatrix(u)
eul = u/180*pi;
rotm = eul2rotm(eul',"XYZ");
end
